simulink model "ASTRA_FES_Simulator"  (R2018b)
settings: Solver=ode5  StartTime=0.0  StopTime=12000  FixedStep=0.01  RelTol=1e-3
values from neighbouring files (symbols this model uses):
  Fail_variance = 0.4/3    (= 0.133333333333)    [ASTRA_FES_Simulator_initialize.m]
undefined symbols (not defined in the file or in its folder): GYRO_sensor_time, lp_gain_GYRO, lp_poles_GYRO, lp_zeros_GYRO, mag_g, mag_h, MTQ_actuator_time, NTUN_ACTS_PP, NTUN_CTR, NTUN_GUI, NTUN_NAV, NTUN_SENS_PP, R_ecef2eci, r_moon, r_sun, S_TIME_ACTS_PP, S_TIME_CTR, S_TIME_GUI, S_TIME_NAV, S_TIME_SENS_PP, tt_s, TUN_ACTS_PP, TUN_CTR, TUN_GUI, TUN_NAV, TUN_SENS_PP
libraries: ENV_Library x9, DKE_Library x4, actuator_library x1, sensor_library x1
settings Model: SimulationMode=accelerator  ExtModeTrigDuration=100  Creator=Andrea  LastModifiedBy=andrea
settings DataIOCC: SaveOutput=off  StateSaveName=tmp_raccel_xout  SignalLoggingName=tmp_raccel_logsout
settings OptimizationCC: EfficientMapNaN2IntZero=off
settings DebuggingCC: AlgebraicLoopMsg=none  ParameterPrecisionLossMsg=none
settings HardwareCC: TargetBitPerLong=64  TargetBitPerPointer=64  TargetBitPerSizeT=64  TargetBitPerPtrDiffT=64  TargetLongLongMode=on  TargetIntDivRoundTo=Zero  TargetEndianess=LittleEndian  TargetWordSize=64  TargetHWDeviceType=MATLAB Host  ProdEqTarget=off
settings ModelReferenceCC: ModelReferenceMinAlgLoopOccurrences=on
settings SFSimCC: SimUseLocalCustomCode=off
settings CodeAppCC: MaxIdLength=128
settings GRTTargetCC: TargetLangStandard=C89/C90 (ANSI)  CombineOutputUpdateFcns=off  GRTInterface=on

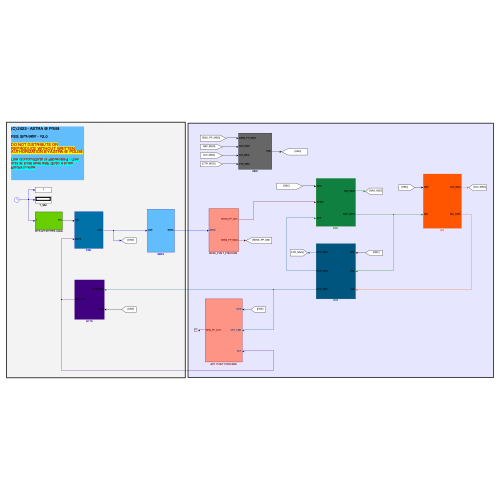
[thumbnail: Simulink's stored preview of the top-level diagram]
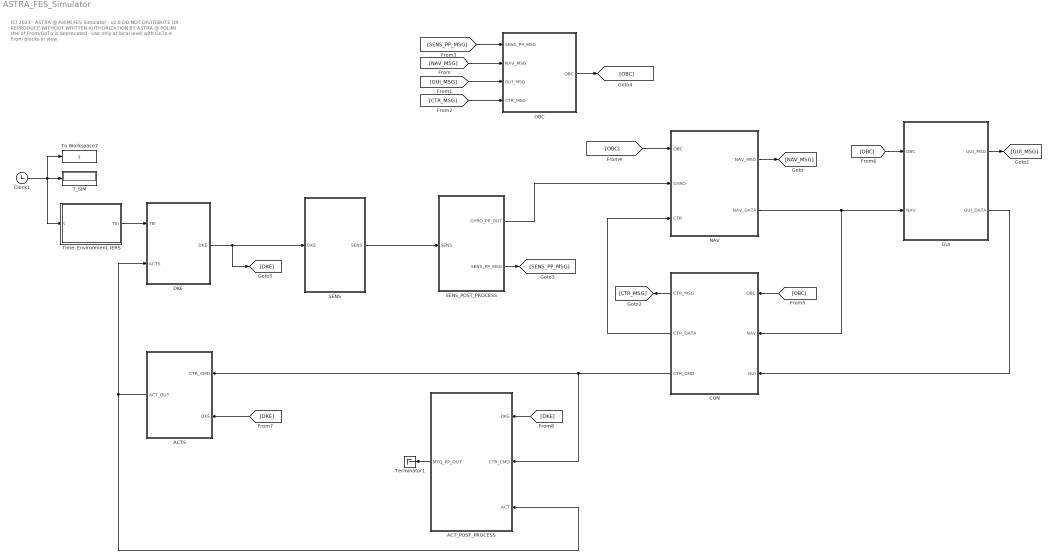
== system ASTRA_FES_Simulator ==
  note: (C) 2023 - ASTRA @ PoliMi
      |
      | FES Simulator - v2.0
      |
      | DO NOT DISTRIBUTE OR REPRODUCE WITHOUT WRITTEN AUTHORIZATION BY ASTRA @ POLIMI
      |
      | Use of From/GoTo is deprecated - Use only at local level with GoTo e From blocks in view
  ACTS : Subsystem
  ACT_POST_PROCESS : Subsystem
  CON : Subsystem
  Clock1 : Clock
  DKE : Subsystem
  GUI : Subsystem
  NAV : Subsystem
  OBC : Subsystem
  SENS : Subsystem
  "SENS_POST_PROCESS " : Subsystem
  T_SIM : Display
  Terminator1 : Terminator
  "Time, Environment, IERS" : Subsystem
  To Workspace7 : ToWorkspace  VariableName=t  SampleTime=-1
  wires:
  Clock1/1 -> "Time, Environment, IERS"/1(t), To Workspace7/1, T_SIM/1
  DKE/1(DKE) -> SENS/1(DKE), [DKE]
  SENS/1(SENS) -> "SENS_POST_PROCESS "/1(SENS)
  "SENS_POST_PROCESS "/1(GYRO_PP_OUT) -> NAV/2(GYRO)
  NAV/1(NAV_MSG) -> [NAV_MSG]
  NAV/2(NAV_DATA) -> CON/2(NAV), GUI/2(NAV)
  CON/3(CTR_CMD) -> ACT_POST_PROCESS/2(CTR_CMD), ACTS/1(CTR_CMD)
  ACTS/1(ACT_OUT) -> DKE/2(ACTS), ACT_POST_PROCESS/3(ACT)
  GUI/2(GUI_DATA) -> CON/3(GUI)
  [NAV_MSG] -> OBC/2(NAV_MSG)
  GUI/1(GUI_MSG) -> [GUI_MSG]
  [GUI_MSG] -> OBC/3(GUI_MSG)
  CON/1(CTR_MSG) -> [CTR_MSG]
  [CTR_MSG] -> OBC/4(CTR_MSG)
  "SENS_POST_PROCESS "/2(SENS_PP_MSG) -> [SENS_PP_MSG]
  [SENS_PP_MSG] -> OBC/1(SENS_PP_MSG)
  ACT_POST_PROCESS/1(MTQ_PP_OUT) -> Terminator1/1
  OBC/1(OBC) -> [OBC]
  [OBC] -> NAV/1(OBC)
  [OBC] -> CON/1(OBC)
  [OBC] -> GUI/1(OBC)
  [DKE] -> ACTS/2(DKE)
  [DKE] -> ACT_POST_PROCESS/1(DKE)
  CON/2(CTR_DATA) -> NAV/3("CTR ")
  "Time, Environment, IERS"/1(TEI) -> DKE/1(TEI)

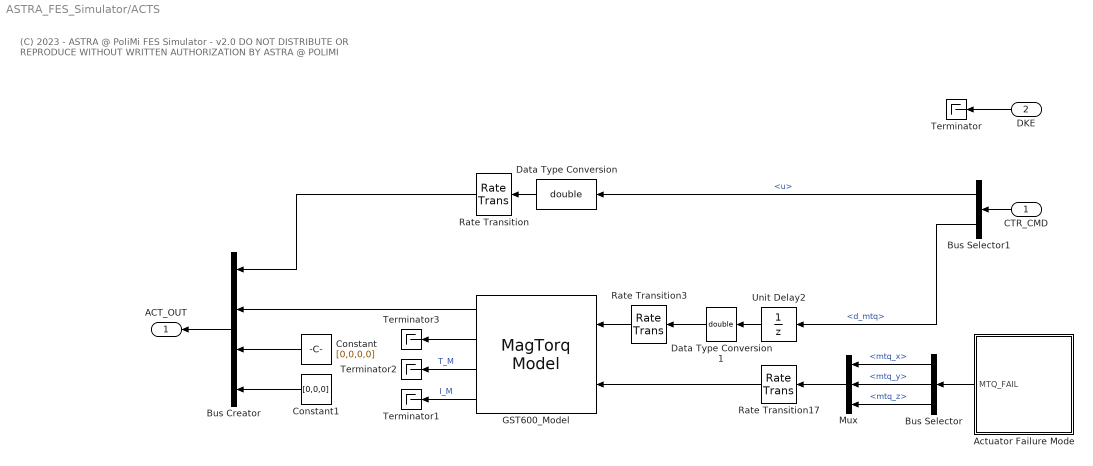
== system ASTRA_FES_Simulator/ACTS ==
  note: (C) 2023 - ASTRA @ PoliMi
      |
      | FES Simulator - v2.0
      |
      | DO NOT DISTRIBUTE OR REPRODUCE WITHOUT WRITTEN AUTHORIZATION BY ASTRA @ POLIMI
  CTR_CMD : Inport  OutDataTypeStr=Bus: CTR_CMD_OUT
  DKE : Inport  Port=2
  Actuator Failure Mode : Subsystem
  Bus Creator : BusCreator  Inputs=4  OutDataTypeStr=Bus: ACTS_OUT
      settings: InheritFromInputs=off
  Bus Selector : BusSelector  OutputSignals=mtq_x,mtq_y,mtq_z
  Bus Selector1 : BusSelector  OutputSignals=u,d_mtq
  Constant : Constant  Value=[0,0,0,0]
  Constant1 : Constant  Value=[0,0,0]
  Data Type Conversion : DataTypeConversion  OutDataTypeStr=double
  Data Type Conversion1 : DataTypeConversion  OutDataTypeStr=double
  GST600_Model : actuator_library/MagTorq Model  mtq=MTQ_DKE  simstep=MTQ_actuator_time
  Mux : Mux  Inputs=3
  Rate Transition : RateTransition  OutPortSampleTime=THR_actuator_time
  Rate Transition17 : RateTransition  OutPortSampleTime=MTQ_actuator_time
  Rate Transition3 : RateTransition  OutPortSampleTime=MTQ_actuator_time
  Terminator{,1..3} (4 alike) : Terminator
  Unit Delay2 : UnitDelay  SampleTime=MTQ_actuator_time  HasFrameUpgradeWarning=on
  ACT_OUT : Outport  OutDataTypeStr=Bus: ACTS_OUT  VectorParamsAs1DForOutWhenUnconnected=off
  wires:
  Unit Delay2/1 -> Data Type Conversion1/1
  Data Type Conversion1/1 -> Rate Transition3/1
  Rate Transition17/1 -> GST600_Model/2
  Mux/1 -> Rate Transition17/1
  Rate Transition3/1 -> GST600_Model/1
  Bus Selector/3 -> Mux/3  "<mtq_z>"
  Bus Selector/2 -> Mux/2  "<mtq_y>"
  Bus Selector/1 -> Mux/1  "<mtq_x>"
  Actuator Failure Mode/1(MTQ_FAIL) -> Bus Selector/1
  DKE/1 -> Terminator/1
  GST600_Model/4 -> Terminator1/1  "I_M"
  GST600_Model/3 -> Terminator2/1  "T_M"
  GST600_Model/2 -> Terminator3/1
  Bus Creator/1 -> ACT_OUT/1
  CTR_CMD/1 -> Bus Selector1/1
  GST600_Model/1 -> Bus Creator/2
  Bus Selector1/2 -> Unit Delay2/1  "<d_mtq>"
  Constant/1 -> Bus Creator/3
  Constant1/1 -> Bus Creator/4
  Bus Selector1/1 -> Data Type Conversion/1  "<u>"
  Data Type Conversion/1 -> Rate Transition/1
  Rate Transition/1 -> Bus Creator/1

== system ASTRA_FES_Simulator/ACT_POST_PROCESS ==
  note: ACT POST PROCESSING BLOCK
  DKE : Inport  OutDataTypeStr=Bus: DKE_OUT
  CTR_CMD : Inport  Port=2  OutDataTypeStr=Bus: CTR_CMD_OUT
  ACT : Inport  Port=3  OutDataTypeStr=Bus: ACTS_OUT
  Bus Creator : BusCreator  Inputs=1  OutDataTypeStr=Bus: ACTS_PP_MTQ_IN
  Bus Selector : BusSelector  OutputSignals=d_mtq
  Rate Transition2 : RateTransition  OutPortSampleTime=S_TIME_ACTS_PP.time_1
  Terminator : Terminator
  Terminator2 : Terminator
  YOUR PP FUNCTION (MTQ AS EXAMPLE) : Subsystem  TreatAsAtomicUnit=on  SystemSampleTime=S_TIME_ACTS_PP.time_1  mask{TUN=TUN_ACTS_PP, NTUN=NTUN_ACTS_PP}
      mask prompts: TUN "Tunable Parameters Structure"; NTUN "NON-Tunable Parameters Structure"
      mask help:
      | % PUT A DESCRIPTION OF THE BLOCK HERE
      |
      | % LIST INPUT DATA
      | % LIST OUTPUT DATA
      | % DEFINE PARAMETERS NAME
      |
      | (c) ASTRA PoliMi - 2023
  MTQ_PP_OUT : Outport  OutDataTypeStr=Bus: ACTS_PP_MTQ_OUT  VectorParamsAs1DForOutWhenUnconnected=off
  wires:
  YOUR PP FUNCTION (MTQ AS EXAMPLE)/1(MTQ_OUT) -> MTQ_PP_OUT/1
  ACT/1 -> Terminator2/1
  DKE/1 -> Terminator/1
  CTR_CMD/1 -> Bus Selector/1
  Bus Selector/1 -> Rate Transition2/1  "<d_mtq>"
  Bus Creator/1 -> YOUR PP FUNCTION (MTQ AS EXAMPLE)/1(MTQ_IN)
  Rate Transition2/1 -> Bus Creator/1  "d_mtq"

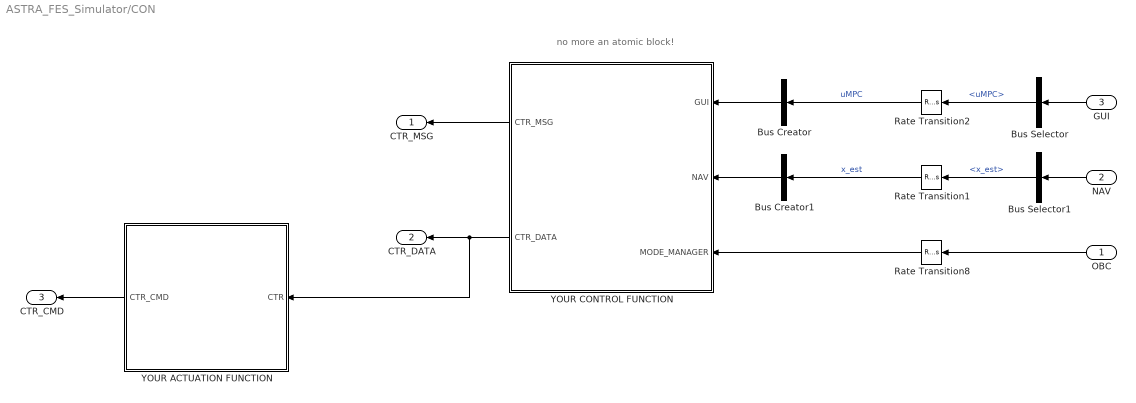
== system ASTRA_FES_Simulator/CON ==
  note: no more an atomic block!
  OBC : Inport  OutDataTypeStr=Bus: OBC_1_OUT
  NAV : Inport  Port=2  OutDataTypeStr=Bus: NAV_DATA_OUT
  GUI : Inport  Port=3  OutDataTypeStr=Bus: GUI_DATA_OUT
  Bus Creator : BusCreator  Inputs=1  OutDataTypeStr=Bus: CTR_GUI_IN
  Bus Creator1 : BusCreator  Inputs=1  OutDataTypeStr=Bus: CTR_NAV_IN
  Bus Selector : BusSelector  OutputSignals=uMPC
  Bus Selector1 : BusSelector  OutputSignals=x_est
  Rate Transition1 : RateTransition  OutPortSampleTime=S_TIME_CTR.time_1
  Rate Transition2 : RateTransition  OutPortSampleTime=S_TIME_CTR.time_2
  Rate Transition8 : RateTransition  OutPortSampleTime=S_TIME_CTR.time_1
  YOUR ACTUATION FUNCTION : Subsystem  TreatAsAtomicUnit=on  SystemSampleTime=S_TIME_CTR.time_1  mask{TUN=TUN_CTR, NTUN=NTUN_CTR}
      mask prompts: TUN "Tunable Parameters Structure"; NTUN "NON-Tunable Parameters Structure"
      mask help:
      | % PUT A DESCRIPTION OF THE BLOCK HERE
      |
      | % LIST INPUT DATA
      | % LIST OUTPUT DATA
      | % DEFINE PARAMETERS NAME
      |
      | (c) ASTRA PoliMi - 2023
  YOUR CONTROL FUNCTION : Subsystem  SystemSampleTime=S_TIME_CTR.time_1  mask{TUN=TUN_NAV, NTUN=NTUN_NAV}
      mask prompts: TUN "Tunable Parameters Structure"; NTUN "NON-Tunable Parameters Structure"
      mask help:
      | % PUT A DESCRIPTION OF THE BLOCK HERE
      |
      | % LIST INPUT DATA
      | % LIST OUTPUT DATA
      | % DEFINE PARAMETERS NAME
      |
      | (c) ASTRA PoliMi - 2023
  CTR_MSG : Outport  OutDataTypeStr=Bus: CTR_MSG_OUT  VectorParamsAs1DForOutWhenUnconnected=off
  CTR_DATA : Outport  Port=2  OutDataTypeStr=Bus: CTR_DATA_OUT  VectorParamsAs1DForOutWhenUnconnected=off
  CTR_CMD : Outport  Port=3  OutDataTypeStr=Bus: CTR_CMD_OUT  VectorParamsAs1DForOutWhenUnconnected=off
  wires:
  OBC/1 -> Rate Transition8/1
  YOUR CONTROL FUNCTION/1(CTR_MSG) -> CTR_MSG/1
  NAV/1 -> Bus Selector1/1
  Rate Transition1/1 -> Bus Creator1/1  "x_est"
  YOUR ACTUATION FUNCTION/1(CTR_CMD) -> CTR_CMD/1
  Rate Transition8/1 -> YOUR CONTROL FUNCTION/3(MODE_MANAGER)
  GUI/1 -> Bus Selector/1
  Bus Creator/1 -> YOUR CONTROL FUNCTION/1(GUI)
  YOUR CONTROL FUNCTION/2(CTR_DATA) -> CTR_DATA/1, YOUR ACTUATION FUNCTION/1(CTR)
  Bus Selector/1 -> Rate Transition2/1  "<uMPC>"
  Rate Transition2/1 -> Bus Creator/1  "uMPC"
  Bus Selector1/1 -> Rate Transition1/1  "<x_est>"
  Bus Creator1/1 -> YOUR CONTROL FUNCTION/2(NAV)

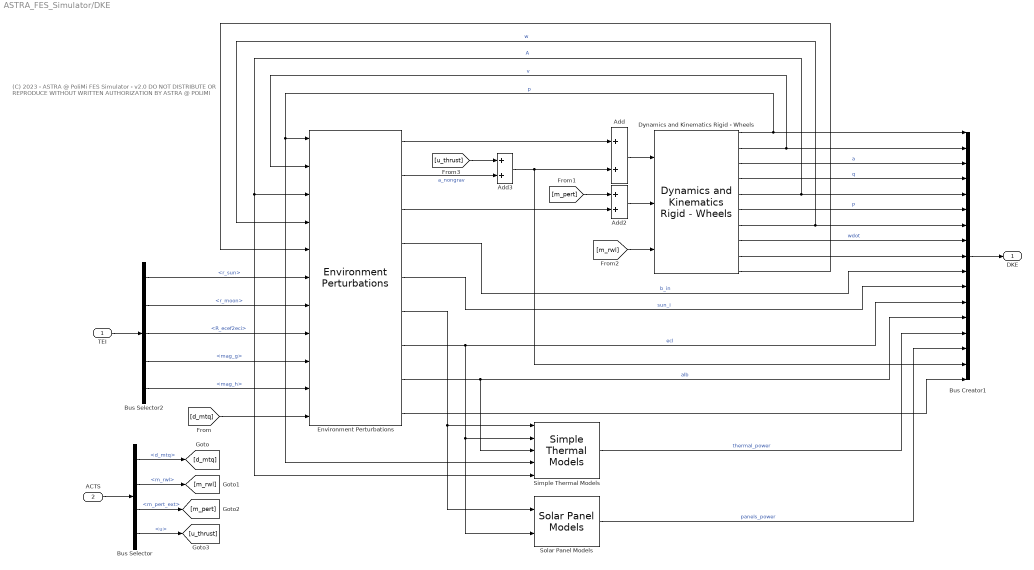
== system ASTRA_FES_Simulator/DKE ==
  note: (C) 2023 - ASTRA @ PoliMi
      |
      | FES Simulator - v2.0
      |
      | DO NOT DISTRIBUTE OR REPRODUCE WITHOUT WRITTEN AUTHORIZATION BY ASTRA @ POLIMI
  TEI : Inport  OutDataTypeStr=Bus: TEI_OUT
  ACTS : Inport  Port=2  OutDataTypeStr=Bus: ACTS_OUT
  " Simple Thermal Models" : DKE_Library/ Simple Thermal Models  P0_Sun=sc.P0_Sun  BODY_RADIUS=env.RADIUS_EARTH  S_surf=sc.S_surf  N_surf=sc.N_surf  vf=env.vf
  Add : Sum
  Add2 : Sum
  Add3 : Sum
  Bus Creator1 : BusCreator  Inputs=17  OutDataTypeStr=Bus: DKE_OUT
      settings: InheritFromInputs=off
  Bus Selector : BusSelector  OutputSignals=d_mtq,m_rwl,m_pert_ext,u
  Bus Selector2 : BusSelector  OutputSignals=r_sun,r_moon,R_ecef2eci,mag_g,mag_h
  Dynamics and Kinematics Rigid - Wheels : DKE_Library/Dynamics and Kinematics  Rigid - Wheels  r0=sc.R0  v0=sc.V0  w0=sc.W0  ww0=sc.WW0  q0=sc.Q0  Im=sc.I  InvIm=sc.invI  GM_BODY=env.GM_EARTH  RWL=RWL_DKE
  Environment Perturbations : DKE_Library/Environment Perturbations  GM_EARTH=env.GM_EARTH  GM_MOON=env.GM_MOON  GM_SUN=env.GM_SUN  RADIUS_EARTH=env.RADIUS_EARTH  RADIUS_SUN=env.RADIUS_SUN  ATMO_HEIGHT=env.ATMO_HEIGHT  mag_data=env.mag_data  grav_data=env.grav_data  rho_h=env.rho_h  NS=sc.NS  S_faces=sc.S_surf  N_faces=sc.N_surf  R_faces=sc.R_surf  c_dif=sc.c_dif  c_spe=sc.c_spe  CD=sc.C_D  mass=sc.m_sc  paras_dipole=sc.d  Keddy=sc.Keddy
  Solar Panel Models : DKE_Library/Solar Panel Models  P0_Sun=sc.P0_Sun  eta_panel=sc.eta_panel  Id=sc.Id  S_panels=sc.S_panels
  DKE : Outport  OutDataTypeStr=Bus: DKE_OUT  VectorParamsAs1DForOutWhenUnconnected=off
  wires:
  ACTS/1 -> Bus Selector/1
  Bus Selector/1 -> [d_mtq]  "<d_mtq>"
  Bus Selector/2 -> [m_rwl]  "<m_rwl>"
  Bus Selector/3 -> [m_pert]  "<m_pert_ext>"
  Bus Selector/4 -> [u_thrust]  "<u>"
  Environment Perturbations/9 -> Bus Creator1/17
  TEI/1 -> Bus Selector2/1
  Environment Perturbations/6 -> Solar Panel Models/1, " Simple Thermal Models"/1
  Environment Perturbations/1 -> Add/1
  Add/1 -> Dynamics and Kinematics Rigid - Wheels/1
  Bus Creator1/1 -> DKE/1
  [m_rwl] -> Dynamics and Kinematics Rigid - Wheels/3
  Environment Perturbations/3 -> Add2/2
  Add2/1 -> Dynamics and Kinematics Rigid - Wheels/2
  [m_pert] -> Add2/1
  Environment Perturbations/2 -> Add3/2  "a_nongrav"
  [u_thrust] -> Add3/1
  Add3/1 -> Bus Creator1/16, Add/2
  Dynamics and Kinematics Rigid - Wheels/1 -> " Simple Thermal Models"/4, Environment Perturbations/1, Bus Creator1/1  "p"
  Dynamics and Kinematics Rigid - Wheels/2 -> Environment Perturbations/2, Bus Creator1/2  "v"
  Dynamics and Kinematics Rigid - Wheels/3 -> Bus Creator1/3  "a"
  Dynamics and Kinematics Rigid - Wheels/4 -> Bus Creator1/4  "q"
  Dynamics and Kinematics Rigid - Wheels/5 -> " Simple Thermal Models"/5, Environment Perturbations/3, Bus Creator1/5  "A"
  Dynamics and Kinematics Rigid - Wheels/6 -> Bus Creator1/6  "P"
  Dynamics and Kinematics Rigid - Wheels/7 -> Bus Creator1/7, Environment Perturbations/4  "w"
  Dynamics and Kinematics Rigid - Wheels/8 -> Bus Creator1/8  "wdot"
  Dynamics and Kinematics Rigid - Wheels/9 -> Bus Creator1/9
  Environment Perturbations/4 -> Bus Creator1/10  "b_in"
  Environment Perturbations/5 -> Bus Creator1/11  "sun_i"
  Environment Perturbations/7 -> Bus Creator1/12, " Simple Thermal Models"/2, Solar Panel Models/2  "ecl"
  Environment Perturbations/8 -> Bus Creator1/13, " Simple Thermal Models"/3  "alb"
  " Simple Thermal Models"/1 -> Bus Creator1/14  "thermal_power"
  Solar Panel Models/1 -> Bus Creator1/15  "panels_power"
  Dynamics and Kinematics Rigid - Wheels/10 -> Environment Perturbations/5
  Bus Selector2/1 -> Environment Perturbations/6  "<r_sun>"
  Bus Selector2/2 -> Environment Perturbations/7  "<r_moon>"
  Bus Selector2/3 -> Environment Perturbations/8  "<R_ecef2eci>"
  Bus Selector2/4 -> Environment Perturbations/9  "<mag_g>"
  Bus Selector2/5 -> Environment Perturbations/10  "<mag_h>"
  [d_mtq] -> Environment Perturbations/11

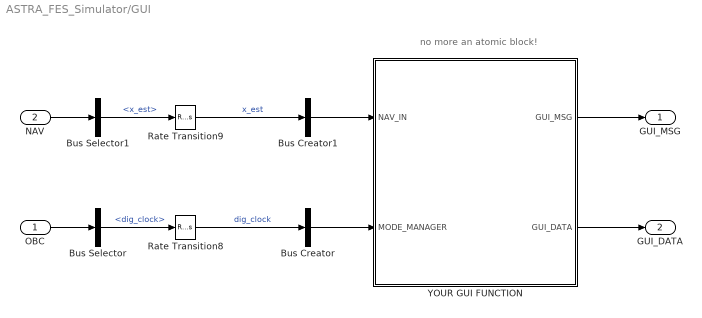
== system ASTRA_FES_Simulator/GUI ==
  note: no more an atomic block!
  OBC : Inport  OutDataTypeStr=Bus: OBC_1_OUT
  NAV : Inport  Port=2  OutDataTypeStr=Bus: NAV_DATA_OUT
  Bus Creator : BusCreator  Inputs=1  OutDataTypeStr=Bus: GUI_MM_IN
  Bus Creator1 : BusCreator  Inputs=1  OutDataTypeStr=Bus: GUI_NAV_IN
  Bus Selector : BusSelector  OutputSignals=dig_clock
  Bus Selector1 : BusSelector  OutputSignals=x_est
  Rate Transition8 : RateTransition  OutPortSampleTime=S_TIME_GUI.time_1
  Rate Transition9 : RateTransition  OutPortSampleTime=S_TIME_GUI.time_1
  YOUR GUI FUNCTION : Subsystem  SystemSampleTime=S_TIME_GUI.time_1  mask{TUN=TUN_GUI, NTUN=NTUN_GUI}
      mask prompts: TUN "Tunable Parameters Structure"; NTUN "NON-Tunable Parameters Structure"
      mask help:
      | % PUT A DESCRIPTION OF THE BLOCK HERE
      |
      | % LIST INPUT DATA
      | % LIST OUTPUT DATA
      | % DEFINE PARAMETERS NAME
      |
      | (c) ASTRA PoliMi - 2023
  GUI_MSG : Outport  OutDataTypeStr=Bus: GUI_MSG_OUT  VectorParamsAs1DForOutWhenUnconnected=off
  GUI_DATA : Outport  Port=2  OutDataTypeStr=Bus: GUI_DATA_OUT  VectorParamsAs1DForOutWhenUnconnected=off
  wires:
  YOUR GUI FUNCTION/2(GUI_DATA) -> GUI_DATA/1
  Bus Creator1/1 -> YOUR GUI FUNCTION/1(NAV_IN)
  YOUR GUI FUNCTION/1(GUI_MSG) -> GUI_MSG/1
  OBC/1 -> Bus Selector/1
  Bus Selector/1 -> Rate Transition8/1  "<dig_clock>"
  Bus Creator/1 -> YOUR GUI FUNCTION/2(MODE_MANAGER)
  NAV/1 -> Bus Selector1/1
  Bus Selector1/1 -> Rate Transition9/1  "<x_est>"
  Rate Transition9/1 -> Bus Creator1/1  "x_est"
  Rate Transition8/1 -> Bus Creator/1  "dig_clock"

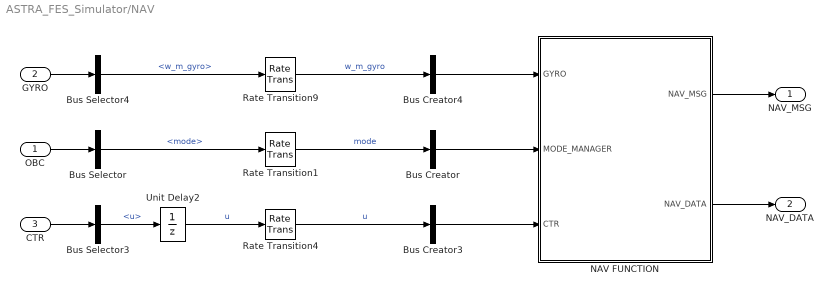
== system ASTRA_FES_Simulator/NAV ==
  OBC : Inport  OutDataTypeStr=Bus: OBC_1_OUT
  GYRO : Inport  Port=2  OutDataTypeStr=Bus: SENS_PP_GYRO_OUT
  "CTR " : Inport  Port=3  OutDataTypeStr=Bus: CTR_DATA_OUT
  Bus Creator : BusCreator  Inputs=1  OutDataTypeStr=Bus: NAV_MM_IN
  Bus Creator3 : BusCreator  Inputs=1  OutDataTypeStr=Bus: NAV_CTR_IN
  Bus Creator4 : BusCreator  Inputs=1  OutDataTypeStr=Bus: NAV_GYRO_IN
  Bus Selector : BusSelector  OutputSignals=mode
  Bus Selector3 : BusSelector  OutputSignals=u
  Bus Selector4 : BusSelector  OutputSignals=w_m_gyro
  NAV FUNCTION : Subsystem  TreatAsAtomicUnit=on  SystemSampleTime=S_TIME_NAV.time_1  mask{TUN=TUN_NAV, NTUN=NTUN_NAV}
      mask prompts: TUN "Tunable Parameters Structure"; NTUN "NON-Tunable Parameters Structure"
      mask help:
      | % PUT A DESCRIPTION OF THE BLOCK HERE
      |
      | % LIST INPUT DATA
      | % LIST OUTPUT DATA
      | % DEFINE PARAMETERS NAME
      |
      | (c) ASTRA PoliMi - 2023
  Rate Transition1 : RateTransition  OutPortSampleTime=S_TIME_NAV.time_1
  Rate Transition4 : RateTransition  OutPortSampleTime=S_TIME_NAV.time_1
  Rate Transition9 : RateTransition  OutPortSampleTime=S_TIME_NAV.time_1
  Unit Delay2 : UnitDelay  InitialCondition=zeros(3, 1)  SampleTime=S_TIME_NAV.time_1  HasFrameUpgradeWarning=on
  NAV_MSG : Outport  OutDataTypeStr=Bus: NAV_MSG_OUT  VectorParamsAs1DForOutWhenUnconnected=off
  NAV_DATA : Outport  Port=2  OutDataTypeStr=Bus: NAV_DATA_OUT  VectorParamsAs1DForOutWhenUnconnected=off
  wires:
  GYRO/1 -> Bus Selector4/1
  OBC/1 -> Bus Selector/1
  NAV FUNCTION/1(NAV_MSG) -> NAV_MSG/1
  Bus Creator/1 -> NAV FUNCTION/2(MODE_MANAGER)
  Bus Creator4/1 -> NAV FUNCTION/1(GYRO)
  NAV FUNCTION/2(NAV_DATA) -> NAV_DATA/1
  Bus Selector/1 -> Rate Transition1/1  "<mode>"
  Bus Creator3/1 -> NAV FUNCTION/3(CTR)
  "CTR "/1 -> Bus Selector3/1
  Bus Selector3/1 -> Unit Delay2/1  "<u>"
  Unit Delay2/1 -> Rate Transition4/1  "u"
  Bus Selector4/1 -> Rate Transition9/1  "<w_m_gyro>"
  Rate Transition4/1 -> Bus Creator3/1  "u"
  Rate Transition1/1 -> Bus Creator/1  "mode"
  Rate Transition9/1 -> Bus Creator4/1  "w_m_gyro"

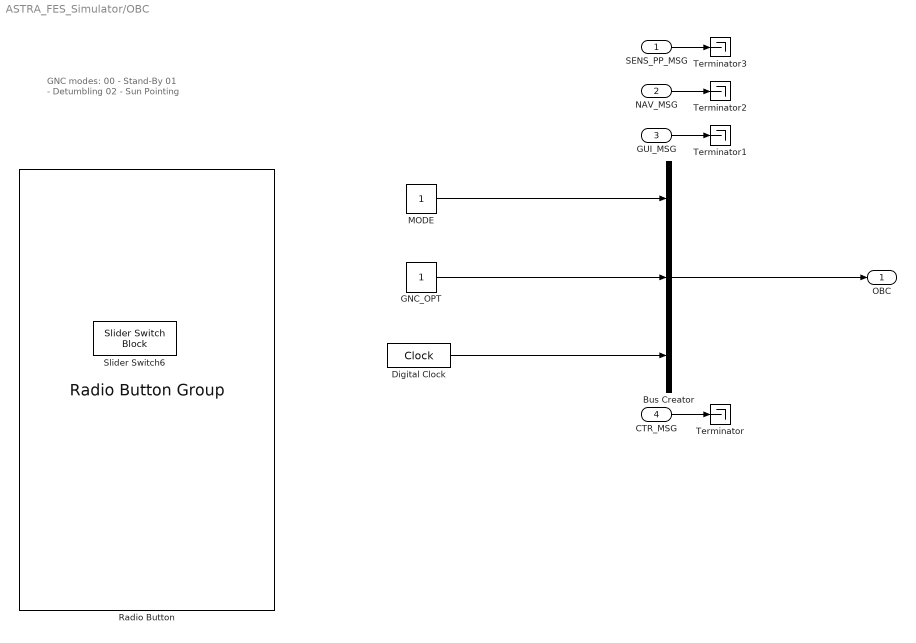
== system ASTRA_FES_Simulator/OBC ==
  note: GNC modes:
      | 00 - Stand-By
      | 01 - Detumbling
      | 02 - Sun Pointing
  SENS_PP_MSG : Inport
  NAV_MSG : Inport  Port=2
  GUI_MSG : Inport  Port=3
  CTR_MSG : Inport  Port=4
  Bus Creator : BusCreator  Inputs=3  OutDataTypeStr=Bus: OBC_1_OUT
      settings: InheritFromInputs=off
  Digital Clock : DigitalClock
  GNC_OPT : Constant  OutDataTypeStr=boolean
  MODE : Constant  OutDataTypeStr=uint16
  Radio Button : RadioButtonGroup  SelectedLabel=Detumbling  ButtonGroupName=Group  WebBlockId=15969
      settings: Values={{'Stand-By', 'Detumbling', 'Sun Pointing'}, [0 1 2]}
  Slider Switch6 : SliderSwitchBlock  WebBlockId=15914
      settings: Values={{'Off', 'On'}, [0 1]}
  Terminator{,1..3} (4 alike) : Terminator
  OBC : Outport  OutDataTypeStr=Bus: OBC_1_OUT  VectorParamsAs1DForOutWhenUnconnected=off
  wires:
  MODE/1 -> Bus Creator/1
  GNC_OPT/1 -> Bus Creator/2
  Bus Creator/1 -> OBC/1
  CTR_MSG/1 -> Terminator/1
  GUI_MSG/1 -> Terminator1/1
  NAV_MSG/1 -> Terminator2/1
  SENS_PP_MSG/1 -> Terminator3/1
  Digital Clock/1 -> Bus Creator/3

== system ASTRA_FES_Simulator/SENS ==
  note: (C) 2023 - ASTRA @ PoliMi
      |
      | FES Simulator - v2.0
      |
      | DO NOT DISTRIBUTE OR REPRODUCE WITHOUT WRITTEN AUTHORIZATION BY ASTRA @ POLIMI
  DKE : Inport  OutDataTypeStr=Bus: DKE_OUT
  Bus Creator1 : BusCreator  Inputs=2  OutDataTypeStr=Bus: SENS_OUT
  Bus Selector2 : BusSelector  OutputSignals=r,q,w
  Sensor Models : Subsystem
  Sensor Reading and Failure Mode : Subsystem
  Sensor Temperature Reading : Subsystem
  To Workspace1 : ToWorkspace  VariableName=q  SampleTime=-1
  To Workspace2 : ToWorkspace  VariableName=w  SampleTime=-1
  To Workspace4 : ToWorkspace  VariableName=r  SampleTime=-1
  SENS : Outport  OutDataTypeStr=Bus: SENS_OUT  VectorParamsAs1DForOutWhenUnconnected=off
  wires:
  Sensor Reading and Failure Mode/1(w_gyro) -> Bus Creator1/1  "w_gyro"
  DKE/1 -> Bus Selector2/1
  Bus Selector2/1 -> To Workspace4/1  "<r>"
  Bus Selector2/2 -> To Workspace1/1  "<q>"
  Bus Selector2/3 -> To Workspace2/1, Sensor Models/1(w_pi)  "<w>"
  Sensor Temperature Reading/1(t_gyro) -> Bus Creator1/2  "t_gyro"
  Bus Creator1/1 -> SENS/1
  Sensor Models/1(w_m_gyro) -> Sensor Reading and Failure Mode/1(w_m_gyro)

== system ASTRA_FES_Simulator/SENS_POST_PROCESS  ==
  note: SENSOR POST PROCESSING BLOCK
  SENS : Inport  OutDataTypeStr=Bus: SENS_OUT
  Bus Creator : BusCreator  Inputs=1  OutDataTypeStr=Bus: SENS_PP_MSG
  Bus Selector : BusSelector  OutputSignals=w_gyro
  Constant : Constant  OutDataTypeStr=uint8
  Rate Transition2 : RateTransition  OutPortSampleTime=S_TIME_SENS_PP.time_1
  YOUR PP FUNCTION (GYRO AS EXAMPLE) : Subsystem  TreatAsAtomicUnit=on  SystemSampleTime=S_TIME_SENS_PP.time_1  mask{TUN=TUN_SENS_PP, NTUN=NTUN_SENS_PP}
      mask prompts: TUN "Tunable Parameters Structure"; NTUN "NON-Tunable Parameters Structure"
      mask help:
      | % PUT A DESCRIPTION OF THE BLOCK HERE
      |
      | % LIST INPUT DATA
      | % LIST OUTPUT DATA
      | % DEFINE PARAMETERS NAME
      |
      | (c) ASTRA PoliMi - 2023
  GYRO_PP_OUT : Outport  OutDataTypeStr=Bus: SENS_PP_GYRO_OUT  VectorParamsAs1DForOutWhenUnconnected=off
  SENS_PP_MSG : Outport  Port=2  OutDataTypeStr=Bus: SENS_PP_MSG  VectorParamsAs1DForOutWhenUnconnected=off
  wires:
  YOUR PP FUNCTION (GYRO AS EXAMPLE)/1(GYRO_M) -> GYRO_PP_OUT/1
  SENS/1 -> Bus Selector/1
  Bus Selector/1 -> Rate Transition2/1  "<w_gyro>"
  Rate Transition2/1 -> YOUR PP FUNCTION (GYRO AS EXAMPLE)/1(w_gyro)
  Constant/1 -> Bus Creator/1  "gyro_error"
  Bus Creator/1 -> SENS_PP_MSG/1

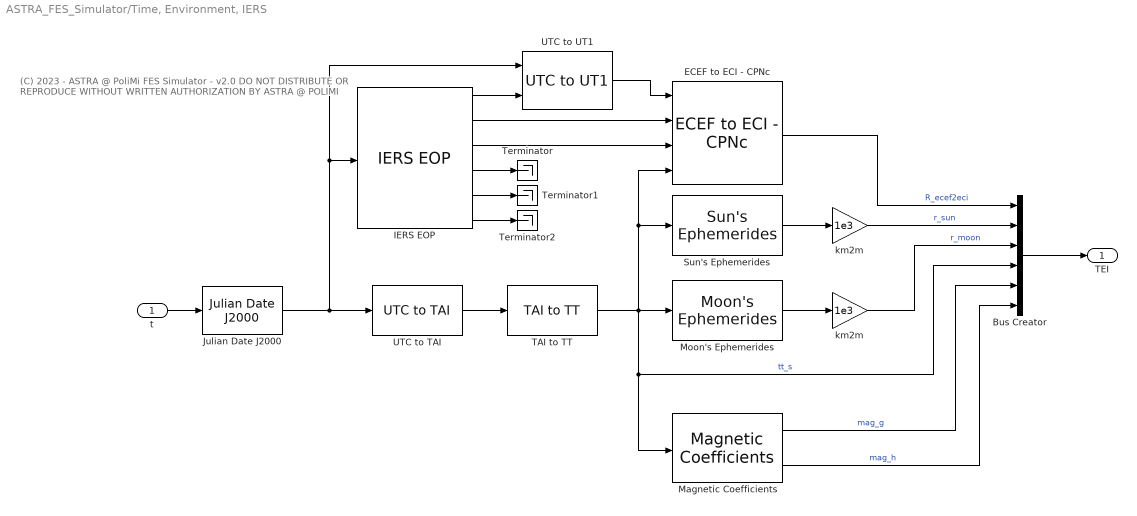
== system ASTRA_FES_Simulator/Time, Environment, IERS ==
  note: (C) 2023 - ASTRA @ PoliMi
      |
      | FES Simulator - v2.0
      |
      | DO NOT DISTRIBUTE OR REPRODUCE WITHOUT WRITTEN AUTHORIZATION BY ASTRA @ POLIMI
  t : Inport
  Bus Creator : BusCreator  Inputs=R_ecef2eci,r_sun,r_moon,tt_s,mag_g,mag_h  OutDataTypeStr=Bus: TEI_OUT
  ECEF to ECI - CPNc : ENV_Library/ECEF to ECI - CPNc
  IERS EOP : ENV_Library/IERS EOP  EOP=env.eop
  Julian Date J2000 : ENV_Library/Julian Date J2000  jd0=env.jdate0
  Magnetic Coefficients : ENV_Library/Magnetic Coefficients  mag_data=env.mag_data
  Moon's Ephemerides : ENV_Library/Moon's Ephemerides
  Sun's Ephemerides : ENV_Library/Sun's Ephemerides
  TAI to TT : ENV_Library/TAI to TT
  Terminator : Terminator
  Terminator1 : Terminator
  Terminator2 : Terminator
  UTC to TAI : ENV_Library/UTC to TAI  leapseconds=env.leap
  UTC to UT1 : ENV_Library/UTC to UT1
  km2m : Gain  Gain=1e3
  "km2m " : Gain  Gain=1e3
  TEI : Outport  OutDataTypeStr=Bus: TEI_OUT  VectorParamsAs1DForOutWhenUnconnected=off
  wires:
  t/1 -> Julian Date J2000/1
  UTC to TAI/1 -> TAI to TT/1
  Julian Date J2000/1 -> UTC to TAI/1, IERS EOP/1, UTC to UT1/1
  TAI to TT/1 -> ECEF to ECI - CPNc/4, Sun's Ephemerides/1, Magnetic Coefficients/1, Bus Creator/4, Moon's Ephemerides/1  "tt_s"
  IERS EOP/1 -> UTC to UT1/2
  UTC to UT1/1 -> ECEF to ECI - CPNc/1
  IERS EOP/4 -> Terminator/1
  IERS EOP/5 -> Terminator1/1
  IERS EOP/6 -> Terminator2/1
  Bus Creator/1 -> TEI/1
  ECEF to ECI - CPNc/1 -> Bus Creator/1  "R_ecef2eci"
  Sun's Ephemerides/1 -> km2m/1
  Moon's Ephemerides/1 -> "km2m "/1
  km2m/1 -> Bus Creator/2  "r_sun"
  "km2m "/1 -> Bus Creator/3  "r_moon"
  IERS EOP/2 -> ECEF to ECI - CPNc/2
  IERS EOP/3 -> ECEF to ECI - CPNc/3
  Magnetic Coefficients/1 -> Bus Creator/5  "mag_g"
  Magnetic Coefficients/2 -> Bus Creator/6  "mag_h"

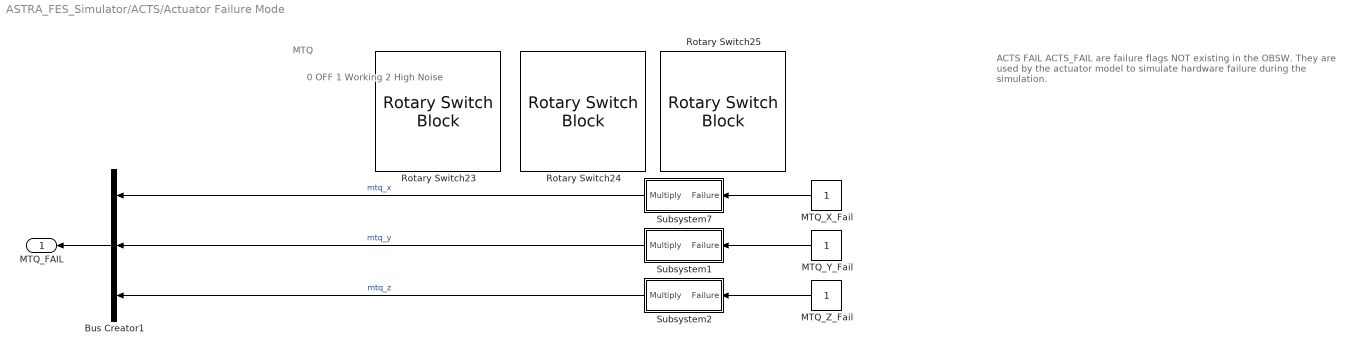
== system ASTRA_FES_Simulator/ACTS/Actuator Failure Mode ==
  note: 0 OFF
      | 1 Working
      | 2 High Noise
  note: MTQ
  note: ACTS FAIL
      |
      | ACTS_FAIL are failure flags NOT existing in the OBSW.
      | They are used by the actuator model to simulate hardware failure during the simulation.
  Bus Creator1 : BusCreator  Inputs=3
  MTQ_X_Fail : Constant  OutDataTypeStr=single  SampleTime=MTQ_actuator_time
  MTQ_Y_Fail : Constant  OutDataTypeStr=single  SampleTime=MTQ_actuator_time
  MTQ_Z_Fail : Constant  OutDataTypeStr=single  SampleTime=MTQ_actuator_time
  Rotary Switch23 : RotarySwitchBlock  WebBlockId=18557
      settings: Values={{'Off', 'Work', 'Noise'}, [0 1 2]}
  Rotary Switch24 : RotarySwitchBlock  WebBlockId=18558
      settings: Values={{'Off', 'Work', 'Noise'}, [0 1 2]}
  Rotary Switch25 : RotarySwitchBlock  WebBlockId=18559
      settings: Values={{'Off', 'Work', 'Noise'}, [0 1 2]}
  Subsystem1 : Subsystem
  Subsystem2 : Subsystem
  Subsystem7 : Subsystem
  MTQ_FAIL : Outport  VectorParamsAs1DForOutWhenUnconnected=off
  wires:
  MTQ_Z_Fail/1 -> Subsystem2/1(Failure)
  MTQ_Y_Fail/1 -> Subsystem1/1(Failure)
  MTQ_X_Fail/1 -> Subsystem7/1(Failure)
  Subsystem2/1(Multiply) -> Bus Creator1/3  "mtq_z"
  Subsystem7/1(Multiply) -> Bus Creator1/1  "mtq_x"
  Subsystem1/1(Multiply) -> Bus Creator1/2  "mtq_y"
  Bus Creator1/1 -> MTQ_FAIL/1

== system ASTRA_FES_Simulator/ACT_POST_PROCESS/YOUR PP FUNCTION (MTQ AS EXAMPLE) ==
  note: ALWAYS FILL DATA TYPE IN INPUT OUTPUT BLOCK. DATA YPE MUST BE A BUS PREVIOUSLY DEFINED.
  note: DEFINE YOUR BUS TYPES
  note: DEFINE YOUR BUS TYPES
  MTQ_IN : Inport  OutDataTypeStr=Bus: ACTS_PP_MTQ_IN
  Bus Creator : BusCreator  Inputs=1  OutDataTypeStr=Bus: ACTS_PP_MTQ_OUT
  Constant : Constant  Value=[1,1,1]  OutDataTypeStr=single
  Terminator : Terminator
  MTQ_OUT : Outport  OutDataTypeStr=Bus: ACTS_PP_MTQ_OUT  VectorParamsAs1DForOutWhenUnconnected=off
  wires:
  MTQ_IN/1 -> Terminator/1
  Bus Creator/1 -> MTQ_OUT/1
  Constant/1 -> Bus Creator/1  "i_mtq"

== system ASTRA_FES_Simulator/CON/YOUR ACTUATION FUNCTION ==
  note: DEFINE YOUR BUS TYPES
  note: DEFINE YOUR BUS TYPES
  note: ALWAYS FILL DATA TYPE IN INPUT OUTPUT BLOCK. DATA YPE MUST BE A BUS PREVIOUSLY DEFINED.
  CTR : Inport  OutDataTypeStr=Bus: CTR_DATA_OUT
  Bus Creator : BusCreator  Inputs=2  OutDataTypeStr=Bus: CTR_CMD_OUT
      settings: InheritFromInputs=off
  Bus Selector : BusSelector  OutputSignals=u
  Constant : Constant  Value=[0,0,0]  OutDataTypeStr=single
  CTR_CMD : Outport  OutDataTypeStr=Bus: CTR_CMD_OUT  VectorParamsAs1DForOutWhenUnconnected=off
  wires:
  Constant/1 -> Bus Creator/1  "d_mtq"
  Bus Creator/1 -> CTR_CMD/1
  CTR/1 -> Bus Selector/1
  Bus Selector/1 -> Bus Creator/2  "<u>"

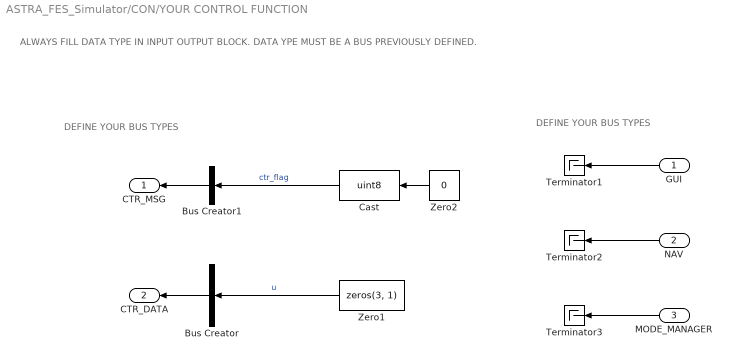
== system ASTRA_FES_Simulator/CON/YOUR CONTROL FUNCTION ==
  note: ALWAYS FILL DATA TYPE IN INPUT OUTPUT BLOCK. DATA YPE MUST BE A BUS PREVIOUSLY DEFINED.
  note: DEFINE YOUR BUS TYPES
  note: DEFINE YOUR BUS TYPES
  GUI : Inport  OutDataTypeStr=Bus: CTR_GUI_IN
  NAV : Inport  Port=2  OutDataTypeStr=Bus: CTR_NAV_IN
  MODE_MANAGER : Inport  Port=3  OutDataTypeStr=Bus: CTR_MM_IN
  Bus Creator : BusCreator  Inputs=1
  Bus Creator1 : BusCreator  Inputs=1
  Cast : DataTypeConversion  OutDataTypeStr=uint8
  Terminator1 : Terminator
  Terminator2 : Terminator
  Terminator3 : Terminator
  Zero1 : Constant  Value=zeros(3, 1)  OutDataTypeStr=single
  Zero2 : Constant  Value=0  OutDataTypeStr=Inherit: Inherit via back propagation
  CTR_MSG : Outport  OutDataTypeStr=Bus: CTR_MSG_OUT  VectorParamsAs1DForOutWhenUnconnected=off
  CTR_DATA : Outport  Port=2  OutDataTypeStr=Bus: CTR_DATA_OUT  VectorParamsAs1DForOutWhenUnconnected=off
  wires:
  Bus Creator/1 -> CTR_DATA/1
  Cast/1 -> Bus Creator1/1  "ctr_flag"
  Bus Creator1/1 -> CTR_MSG/1
  Zero1/1 -> Bus Creator/1  "u"
  GUI/1 -> Terminator1/1
  NAV/1 -> Terminator2/1
  MODE_MANAGER/1 -> Terminator3/1
  Zero2/1 -> Cast/1

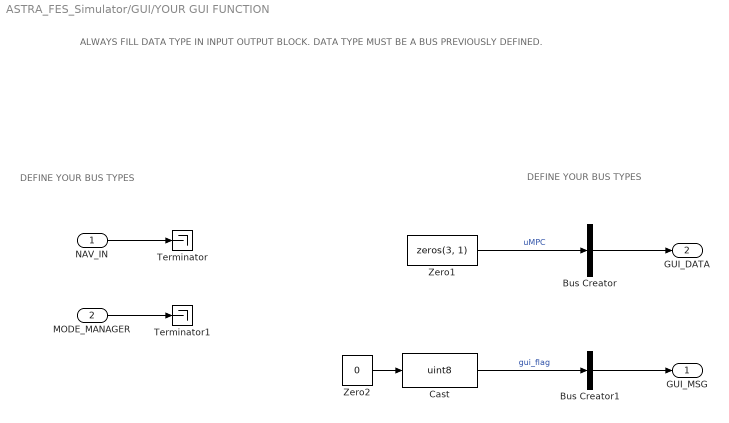
== system ASTRA_FES_Simulator/GUI/YOUR GUI FUNCTION ==
  note: DEFINE YOUR BUS TYPES
  note: DEFINE YOUR BUS TYPES
  note: ALWAYS FILL DATA TYPE IN INPUT OUTPUT BLOCK. DATA TYPE MUST BE A BUS PREVIOUSLY DEFINED.
  NAV_IN : Inport  OutDataTypeStr=Bus: GUI_NAV_IN
  MODE_MANAGER : Inport  Port=2  OutDataTypeStr=Bus: GUI_MM_IN
  Bus Creator : BusCreator  Inputs=1  OutDataTypeStr=Bus: GUI_DATA_OUT
  Bus Creator1 : BusCreator  Inputs=1
  Cast : DataTypeConversion  OutDataTypeStr=uint8
  Terminator : Terminator
  Terminator1 : Terminator
  Zero1 : Constant  Value=zeros(3, 1)  OutDataTypeStr=single
  Zero2 : Constant  Value=0  OutDataTypeStr=Inherit: Inherit via back propagation
  GUI_MSG : Outport  OutDataTypeStr=Bus: GUI_MSG_OUT  VectorParamsAs1DForOutWhenUnconnected=off
  GUI_DATA : Outport  Port=2  OutDataTypeStr=Bus: GUI_DATA_OUT  VectorParamsAs1DForOutWhenUnconnected=off
  wires:
  Bus Creator/1 -> GUI_DATA/1
  Bus Creator1/1 -> GUI_MSG/1
  Zero1/1 -> Bus Creator/1  "uMPC"
  NAV_IN/1 -> Terminator/1
  MODE_MANAGER/1 -> Terminator1/1
  Zero2/1 -> Cast/1
  Cast/1 -> Bus Creator1/1  "gui_flag"

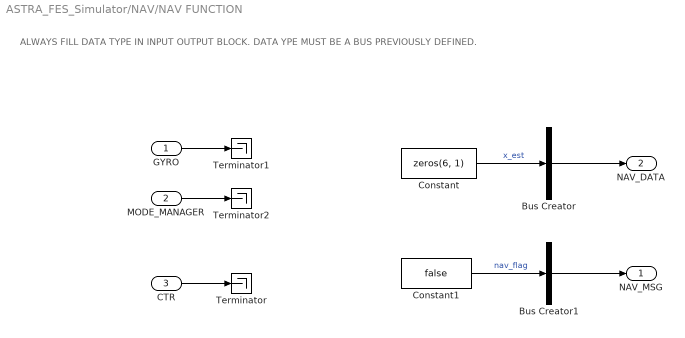
== system ASTRA_FES_Simulator/NAV/NAV FUNCTION ==
  note: ALWAYS FILL DATA TYPE IN INPUT OUTPUT BLOCK. DATA YPE MUST BE A BUS PREVIOUSLY DEFINED.
  GYRO : Inport  OutDataTypeStr=Bus: NAV_GYRO_IN
  MODE_MANAGER : Inport  Port=2  OutDataTypeStr=Bus: NAV_MM_IN
  CTR : Inport  Port=3  OutDataTypeStr=Bus: NAV_CTR_IN
  Bus Creator : BusCreator  Inputs=1  OutDataTypeStr=Bus: NAV_DATA_OUT
  Bus Creator1 : BusCreator  Inputs=1  OutDataTypeStr=Bus: NAV_MSG_OUT
  Constant : Constant  Value=zeros(6, 1)  OutDataTypeStr=single
  Constant1 : Constant  Value=false  OutDataTypeStr=boolean
  Terminator : Terminator
  Terminator1 : Terminator
  Terminator2 : Terminator
  NAV_MSG : Outport  OutDataTypeStr=Bus: NAV_MSG_OUT  VectorParamsAs1DForOutWhenUnconnected=off
  NAV_DATA : Outport  Port=2  OutDataTypeStr=Bus: NAV_DATA_OUT  VectorParamsAs1DForOutWhenUnconnected=off
  wires:
  Bus Creator1/1 -> NAV_MSG/1
  Bus Creator/1 -> NAV_DATA/1
  CTR/1 -> Terminator/1
  GYRO/1 -> Terminator1/1
  MODE_MANAGER/1 -> Terminator2/1
  Constant/1 -> Bus Creator/1  "x_est"
  Constant1/1 -> Bus Creator1/1  "nav_flag"

== system ASTRA_FES_Simulator/SENS/Sensor Models ==
  note: PLACE SENSORS HERE
  note: deg/s
  note: Low pass filters in this block are those contained in the sensor components. NOT in GNC.
  note: rad/s
  w_pi : Inport
  Data Type Conversion2 : DataTypeConversion  OutDataTypeStr=single
  Gyro Model  (deg/s ) : sensor_library/Gyro Model  (deg//s)  gyros=GYRO.gyros  simstep=GYRO_sensor_time
  Omega Filter GYRO : Subsystem  mask(Low Pass Filter (3D)){zeros=lp_zeros_GYRO, poles=lp_poles_GYRO, gain=lp_gain_GYRO, sampletime=GYRO_sensor_time}
      mask prompts: zeros "Filter Zeros"; poles "Filter Poles"; gain "Filter Gain"; sampletime "Filter Sample Time"
      mask help:
      | 3 Dimension Low Pass Filter
      |
      | Input Specifies Gain, Zero, Poles and Sample Time
  w_m_gyro : Outport  VectorParamsAs1DForOutWhenUnconnected=off
  wires:
  Gyro Model  (deg/s )/1 -> Omega Filter GYRO/1(w_m)
  w_pi/1 -> Gyro Model  (deg/s )/1
  Data Type Conversion2/1 -> w_m_gyro/1
  Omega Filter GYRO/1(w_m_f) -> Data Type Conversion2/1

== system ASTRA_FES_Simulator/SENS/Sensor Reading and Failure Mode ==
  note: GYRO
  w_m_gyro : Inport
  GYRO_Fail : Constant  OutDataTypeStr=single  SampleTime=GYRO_sensor_time
  Multiply7 : Product
  Rotary Switch25 : RotarySwitchBlock  WebBlockId=18251
      settings: Values={{'Off', 'Work', 'Noise'}, [0 1 2]}
  Subsystem7 : Subsystem
  w_gyro : Outport  VectorParamsAs1DForOutWhenUnconnected=off
  wires:
  Multiply7/1 -> w_gyro/1
  Subsystem7/1(Multiply) -> Multiply7/2
  GYRO_Fail/1 -> Subsystem7/1(Failure)
  w_m_gyro/1 -> Multiply7/1

== system ASTRA_FES_Simulator/SENS/Sensor Temperature Reading ==
  note: GYRO TEMPERATURE
  Add6 : Sum
  Data Type Conversion : DataTypeConversion  OutDataTypeStr=single
  GYRO : Constant  Value=22  OutDataTypeStr=single  SampleTime=S_TIME_NAV.time_1
  Rotary Switch5 : RotarySwitchBlock  LabelPosition=Hide  WebBlockId=18432
      settings: Values={{'Cold', 'Nominal', 'Hot'}, [-100 22 100]}
  Temperature Oscillations to have NON constant values : Sin  Amplitude=5*ones(1,1)  Bias=0*ones(1,1)  Frequency=0.1*ones(1,1)  Phase=2*pi*randn(1,1)  SampleTime=GYRO_sensor_time
  t_gyro : Outport  VectorParamsAs1DForOutWhenUnconnected=off
  wires:
  GYRO/1 -> Add6/2
  Temperature Oscillations to have NON constant values/1 -> Data Type Conversion/1
  Add6/1 -> t_gyro/1
  Data Type Conversion/1 -> Add6/1

== system ASTRA_FES_Simulator/SENS_POST_PROCESS /YOUR PP FUNCTION (GYRO AS EXAMPLE) ==
  note: ALWAYS FILL DATA TYPE IN INPUT OUTPUT BLOCK. DATA YPE MUST BE A BUS PREVIOUSLY DEFINED.
  note: DEFINE YOUR BUS TYPES
  note: DEFINE YOUR BUS TYPES
  w_gyro : Inport
  Bus Creator : BusCreator  Inputs=1  OutDataTypeStr=Bus: SENS_PP_GYRO_OUT
      settings: InheritFromInputs=off
  GYRO_M : Outport  OutDataTypeStr=Bus: SENS_PP_GYRO_OUT  VectorParamsAs1DForOutWhenUnconnected=off
  wires:
  w_gyro/1 -> Bus Creator/1
  Bus Creator/1 -> GYRO_M/1

== system ASTRA_FES_Simulator/ACTS/Actuator Failure Mode/Subsystem1 ==
  Failure : Inport
  Constant : Constant  Value=0  OutDataTypeStr=single  SampleTime=MTQ_actuator_time
  Constant1 : Constant  OutDataTypeStr=single  SampleTime=MTQ_actuator_time
  Multiport Switch : MultiPortSwitch  DataPortOrder=Zero-based contiguous  zeroidx=on
  Random Number : RandomNumber  Mean=1  Variance=(200*Fail_variance)^2  Seed=82635  SampleTime=MTQ_actuator_time
  Multiply : Outport  VectorParamsAs1DForOutWhenUnconnected=off
  wires:
  Failure/1 -> Multiport Switch/1
  Multiport Switch/1 -> Multiply/1
  Random Number/1 -> Multiport Switch/4
  Constant/1 -> Multiport Switch/2
  Constant1/1 -> Multiport Switch/3

== system ASTRA_FES_Simulator/ACTS/Actuator Failure Mode/Subsystem2 ==
  Failure : Inport
  Constant : Constant  Value=0  OutDataTypeStr=single  SampleTime=MTQ_actuator_time
  Constant1 : Constant  OutDataTypeStr=single  SampleTime=MTQ_actuator_time
  Multiport Switch : MultiPortSwitch  DataPortOrder=Zero-based contiguous  zeroidx=on
  Random Number : RandomNumber  Mean=1  Variance=(200*Fail_variance)^2  Seed=1265126  SampleTime=MTQ_actuator_time
  Multiply : Outport  VectorParamsAs1DForOutWhenUnconnected=off
  wires:
  Constant1/1 -> Multiport Switch/3
  Constant/1 -> Multiport Switch/2
  Random Number/1 -> Multiport Switch/4
  Multiport Switch/1 -> Multiply/1
  Failure/1 -> Multiport Switch/1

== system ASTRA_FES_Simulator/ACTS/Actuator Failure Mode/Subsystem7 ==
  Failure : Inport
  Constant : Constant  Value=0  OutDataTypeStr=single  SampleTime=MTQ_actuator_time
  Constant1 : Constant  OutDataTypeStr=single  SampleTime=MTQ_actuator_time
  Multiport Switch : MultiPortSwitch  DataPortOrder=Zero-based contiguous  zeroidx=on
  Random Number : RandomNumber  Mean=1  Variance=(200*Fail_variance)^2  Seed=875143  SampleTime=MTQ_actuator_time
  Multiply : Outport  VectorParamsAs1DForOutWhenUnconnected=off
  wires:
  Constant1/1 -> Multiport Switch/3
  Constant/1 -> Multiport Switch/2
  Random Number/1 -> Multiport Switch/4
  Multiport Switch/1 -> Multiply/1
  Failure/1 -> Multiport Switch/1

== system ASTRA_FES_Simulator/SENS/Sensor Models/Omega Filter GYRO ==
  w_m : Inport
  Demux1 : Demux  Outputs=3
  Discrete Zero-Pole : DiscreteZeroPole  Zeros=zeros  Poles=poles  Gain=gain  SampleTime=sampletime
  Discrete Zero-Pole1 : DiscreteZeroPole  Zeros=zeros  Poles=poles  Gain=gain  SampleTime=sampletime
  Discrete Zero-Pole2 : DiscreteZeroPole  Zeros=zeros  Poles=poles  Gain=gain  SampleTime=sampletime
  Mux1 : Mux  Inputs=3
  w_m_f : Outport  VectorParamsAs1DForOutWhenUnconnected=off
  wires:
  w_m/1 -> Demux1/1
  Discrete Zero-Pole/1 -> Mux1/1
  Discrete Zero-Pole2/1 -> Mux1/3
  Discrete Zero-Pole1/1 -> Mux1/2
  Demux1/1 -> Discrete Zero-Pole/1
  Mux1/1 -> w_m_f/1
  Demux1/3 -> Discrete Zero-Pole2/1
  Demux1/2 -> Discrete Zero-Pole1/1

== system ASTRA_FES_Simulator/SENS/Sensor Reading and Failure Mode/Subsystem7 ==
  Failure : Inport
  Constant : Constant  Value=0  OutDataTypeStr=single  SampleTime=GYRO_sensor_time
  Constant1 : Constant  OutDataTypeStr=single  SampleTime=GYRO_sensor_time
  Data Type Conversion : DataTypeConversion  OutDataTypeStr=single
  Multiport Switch : MultiPortSwitch  DataPortOrder=Zero-based contiguous  zeroidx=on
  Random Number : RandomNumber  Mean=1  Variance=(50*Fail_variance)^2  Seed=875143  SampleTime=GYRO_sensor_time
  Multiply : Outport  VectorParamsAs1DForOutWhenUnconnected=off
  wires:
  Constant1/1 -> Multiport Switch/3
  Constant/1 -> Multiport Switch/2
  Data Type Conversion/1 -> Multiport Switch/4
  Random Number/1 -> Data Type Conversion/1
  Multiport Switch/1 -> Multiply/1
  Failure/1 -> Multiport Switch/1
